simulink model "HallSensor1"  (R2023a)
settings: Solver=VariableStepAuto  StartTime=0.0  StopTime=10.0  RelTol=1e-3
settings Model: Creator=mrrom  LastModifiedBy=mrrom

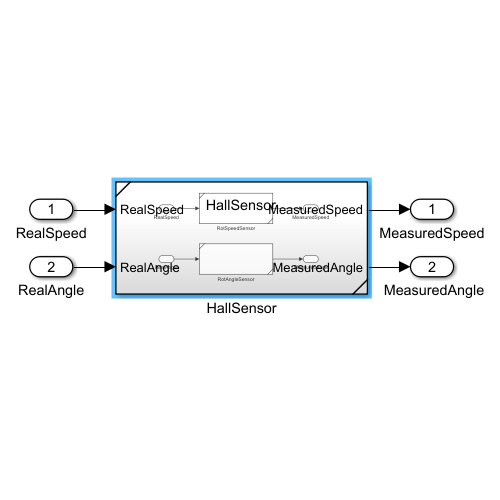
[thumbnail: Simulink's stored preview of the top-level diagram]
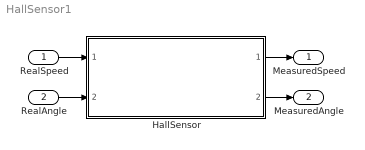
== system HallSensor1 ==
  RealSpeed : Inport
  RealAngle : Inport  Port=2
  HallSensor : Subsystem  ReferencedSubsystem=HallSensor
  MeasuredSpeed : Outport
  " MeasuredAngle" : Outport  Port=2
  wires:
  RealSpeed/1 -> HallSensor/1
  RealAngle/1 -> HallSensor/2
  HallSensor/1 -> MeasuredSpeed/1
  HallSensor/2 -> " MeasuredAngle"/1
